simulink model "ex5_2"  (R2018b)
settings: Solver=VariableStepAuto  StartTime=0.0  StopTime=18  RelTol=1e-3
settings Model: Creator=HYJ  LastModifiedBy=HYJ

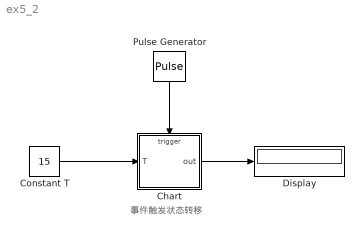
== system ex5_2 ==
  note: 事件触发状态转移
  Chart : Stateflow chart  TreatAsAtomicUnit=on
  Constant T : Constant  Value=15
  Display : Display
  Pulse Generator : DiscretePulseGenerator  PulseType=Time based  Period=10  PulseWidth=5
  wires:
  Constant T/1 -> Chart/1(T)
  Chart/1(out) -> Display/1
  Pulse Generator/1 -> Chart/Trigger

== stateflow chart ex5_2/Chart ==
  state reset
    en: out = 0;
  state count
    en: out = out + 1;
  (default) -> reset
  (junction 12) -> reset [order 1] : [out>=T]
  reset -> (junction 12) : E
  count -> (junction 12) : E
  (junction 12) -> count [order 2] : [out<T]
  data: T input; out output
  events: E input RISING_EDGE_EVENT
